simulink model "DroneDF"  (R2026a)
settings: Solver=VariableStepAuto
settings Model: Creator=Paila  LastModifiedBy=Paila

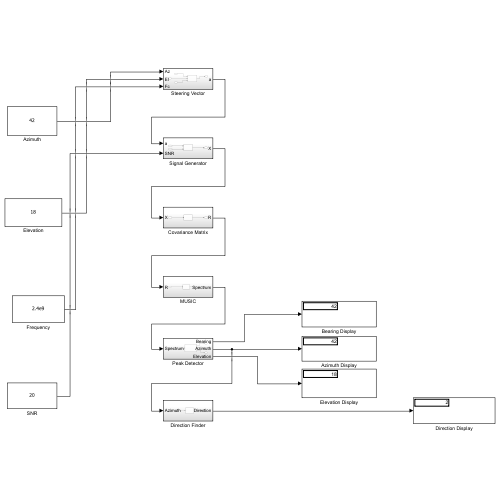
[thumbnail: Simulink's stored preview of the top-level diagram]
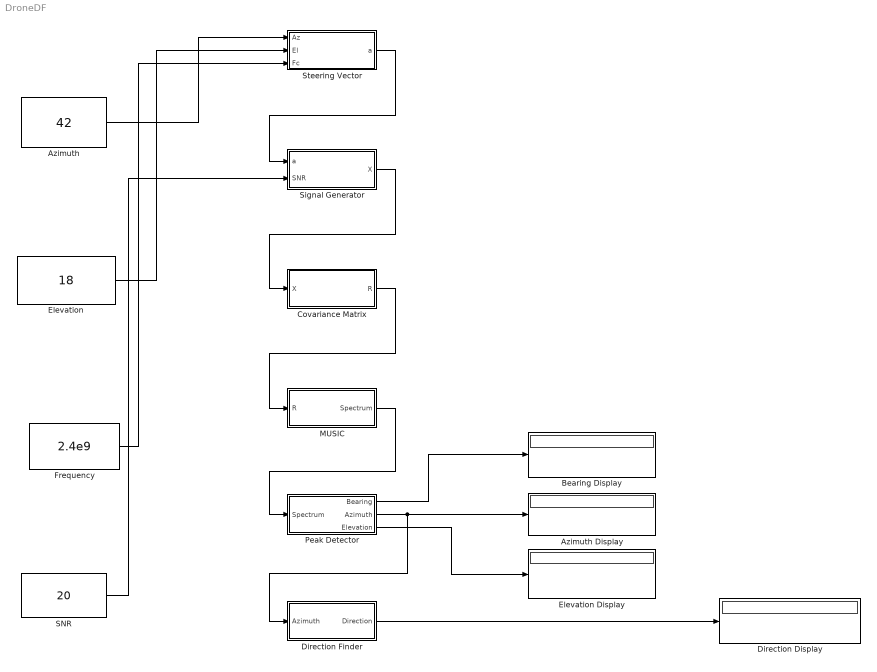
== system DroneDF ==
  Azimuth : Constant  Value=42
  Azimuth Display : Display
  Bearing Display : Display
  Covariance Matrix : Subsystem
  Direction Display : Display
  Direction Finder : Subsystem
  Elevation : Constant  Value=18
  Elevation Display : Display
  Frequency : Constant  Value=2.4e9
  MUSIC : Subsystem
  Peak Detector : Subsystem
  SNR : Constant  Value=20
  Signal Generator : Subsystem
  Steering Vector : Subsystem
  wires:
  Azimuth/1 -> Steering Vector/1(Az)
  Elevation/1 -> Steering Vector/2(El)
  Frequency/1 -> Steering Vector/3(Fc)
  Steering Vector/1(a) -> Signal Generator/1(a)
  SNR/1 -> Signal Generator/2(SNR)
  Signal Generator/1(X) -> Covariance Matrix/1(X)
  Covariance Matrix/1(R) -> MUSIC/1(R)
  MUSIC/1(Spectrum) -> Peak Detector/1(Spectrum)
  Peak Detector/1(Bearing) -> Bearing Display/1
  Peak Detector/2(Azimuth) -> Direction Finder/1(Azimuth), Azimuth Display/1
  Peak Detector/3(Elevation) -> Elevation Display/1
  Direction Finder/1(Direction) -> Direction Display/1

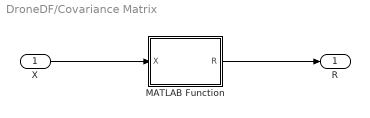
== system DroneDF/Covariance Matrix ==
  X : Inport
  MATLAB Function : MATLAB Function  TreatAsAtomicUnit=on
  R : Outport
  wires:
  X/1 -> MATLAB Function/1(X)
  MATLAB Function/1(R) -> R/1

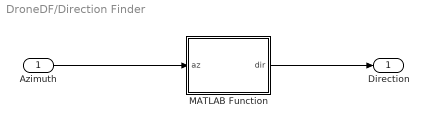
== system DroneDF/Direction Finder ==
  Azimuth : Inport
  MATLAB Function : MATLAB Function  TreatAsAtomicUnit=on
  Direction : Outport
  wires:
  Azimuth/1 -> MATLAB Function/1(az)
  MATLAB Function/1(dir) -> Direction/1

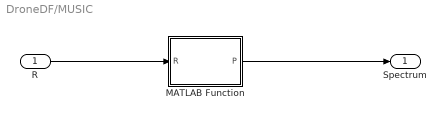
== system DroneDF/MUSIC ==
  R : Inport
  MATLAB Function : MATLAB Function  TreatAsAtomicUnit=on
  Spectrum : Outport
  wires:
  R/1 -> MATLAB Function/1(R)
  MATLAB Function/1(P) -> Spectrum/1

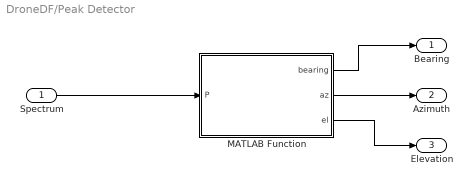
== system DroneDF/Peak Detector ==
  Spectrum : Inport
  MATLAB Function : MATLAB Function  TreatAsAtomicUnit=on
  Bearing : Outport
  Azimuth : Outport  Port=2
  Elevation : Outport  Port=3
  wires:
  Spectrum/1 -> MATLAB Function/1(P)
  MATLAB Function/1(bearing) -> Bearing/1
  MATLAB Function/2(az) -> Azimuth/1
  MATLAB Function/3(el) -> Elevation/1

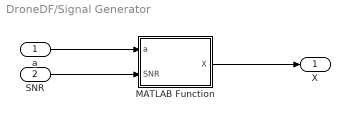
== system DroneDF/Signal Generator ==
  a : Inport
  SNR : Inport  Port=2
  MATLAB Function : MATLAB Function  TreatAsAtomicUnit=on
  X : Outport
  wires:
  a/1 -> MATLAB Function/1(a)
  SNR/1 -> MATLAB Function/2(SNR)
  MATLAB Function/1(X) -> X/1

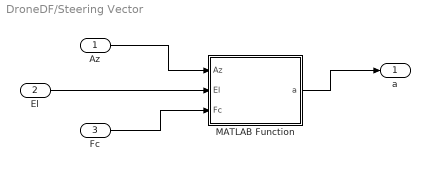
== system DroneDF/Steering Vector ==
  Az : Inport
  El : Inport  Port=2
  Fc : Inport  Port=3
  MATLAB Function : MATLAB Function  TreatAsAtomicUnit=on
  a : Outport
  wires:
  MATLAB Function/1(a) -> a/1
  El/1 -> MATLAB Function/2(El)
  Az/1 -> MATLAB Function/1(Az)
  Fc/1 -> MATLAB Function/3(Fc)

== matlab function DroneDF/Signal Generator/MATLAB Function ==
  data: X output; a input; SNR input
function X = fcn(a,SNR)

snapshots = 1024;

s = randn(1,snapshots);

signal = a*s;

noise = randn(size(signal));

noise = noise ./ norm(noise);

noise = noise .* 10^(-SNR/20);

X = signal + noise;

end

== matlab function DroneDF/Steering Vector/MATLAB Function ==
  data: Az input; a output; El input; Fc input
function a = fcn(Az,El,Fc)

c = 3e8;

lambda = c/Fc;

d = lambda/2;

x = [0 d 0 -d];

y = [d 0 -d 0];

k = 2*pi/lambda;

phase = k*( ...
    x*cosd(El)*cosd(Az) + ...
    y*cosd(El)*sind(Az));

a = exp(1j*phase).';

end

== matlab function DroneDF/Covariance Matrix/MATLAB Function ==
  data: R output; X input
function R = fcn(X)

R = X*X';

R = R/size(X,2);

end

== matlab function DroneDF/MUSIC/MATLAB Function ==
  data: R input; P output
function P = fcn(R)

P = abs(trace(R));

end

== matlab function DroneDF/Peak Detector/MATLAB Function ==
  data: P input; bearing output; az output; el output
function [bearing,az,el] = fcn(P)

% Placeholder detector

az = 42;

el = 18;

bearing = az;

end

== matlab function DroneDF/Direction Finder/MATLAB Function ==
  data: az input; dir output
function dir = fcn(az)

if az >= 337.5 || az < 22.5

    dir = 1;

elseif az < 67.5

    dir = 2;

elseif az < 112.5

    dir = 3;

elseif az < 157.5

    dir = 4;

elseif az < 202.5

    dir = 5;

elseif az < 247.5

    dir = 6;

elseif az < 292.5

    dir = 7;

else

    dir = 8;

end

end
